simulink model "servo"  (R2022a)
settings: Solver=VariableStepAuto  StartTime=0.0  StopTime=15  RelTol=1e-3
values from neighbouring files (symbols this model uses):
  A = [0 0 0 1 0 0 ... (first row only)    [main.m]
  B = [0 0 ... (first row only)    [main.m]
  C = [1 0 0 0 0 0 ... (first row only)    [main.m]
  ka6 = real(inv(R)*Ba6'*P2)    [main.m]
settings Model: Creator=qidon  LastModifiedBy=dzsgy

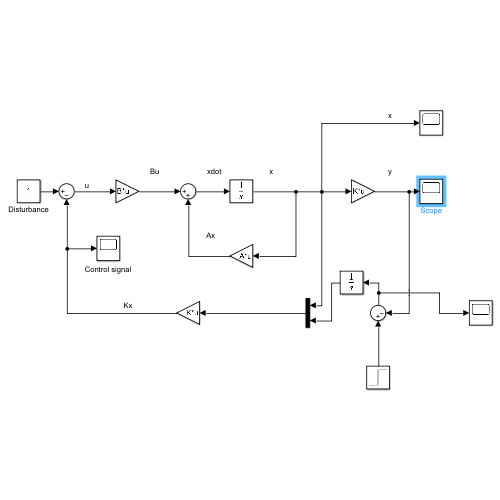
[thumbnail: Simulink's stored preview of the top-level diagram]
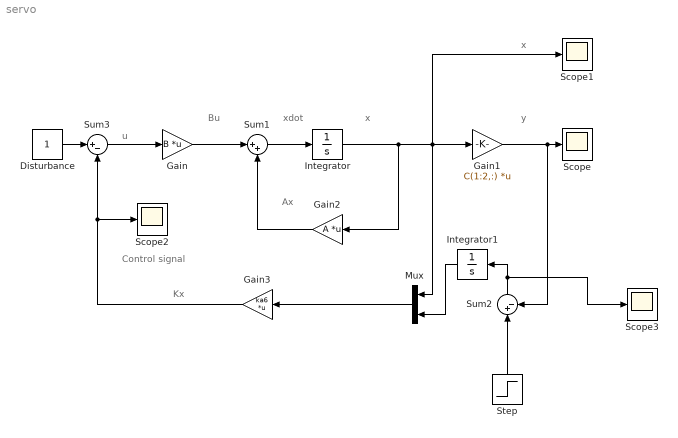
== system servo ==
  note: Kx
  note: x
  note: y
  note: Ax
  note: Bu
  note: x
  note: u
  note: Control signal
  note: xdot
  Disturbance : Constant
  Gain : Gain  Gain=B  Multiplication=Matrix(K*u)
  Gain1 : Gain  Gain=C(1:2,:)  Multiplication=Matrix(K*u)
  Gain2 : Gain  Gain=A  Multiplication=Matrix(K*u)
  Gain3 : Gain  Gain=ka6  Multiplication=Matrix(K*u)
  Integrator : Integrator
  Integrator1 : Integrator
  Mux : Mux  Inputs=2
  Scope{,1..3} (4 alike) : Scope
  Step : Step  After=[1,-0.5]  SampleTime=0
  Sum1 : Sum  Inputs=|++
  Sum2 : Sum  Inputs=|+-
  Sum3 : Sum  Inputs=|+-
  wires:
  Gain3/1 -> Scope2/1, Sum3/2
  Sum3/1 -> Gain/1
  Gain/1 -> Sum1/1
  Sum1/1 -> Integrator/1
  Gain2/1 -> Sum1/2
  Integrator/1 -> Gain2/1, Mux/1, Scope1/1, Gain1/1
  Gain1/1 -> Sum2/2, Scope/1
  Disturbance/1 -> Sum3/1
  Sum2/1 -> Scope3/1, Integrator1/1
  Step/1 -> Sum2/1
  Integrator1/1 -> Mux/2
  Mux/1 -> Gain3/1
